simulink model "electric_vehicle3"  (R2018a)
settings: Solver=VariableStepAuto  StartTime=0.0  StopTime=2474  RelTol=1e-3
undefined symbols (not defined in the file): DiscIntNeverNeededParam
libraries: fl_lib x13, nesl_utility x7, sdl_lib x5, elec_lib x3, autolibshared x2, pe_lib x1
settings Model: Creator=Asus  LastModifiedBy=Asus

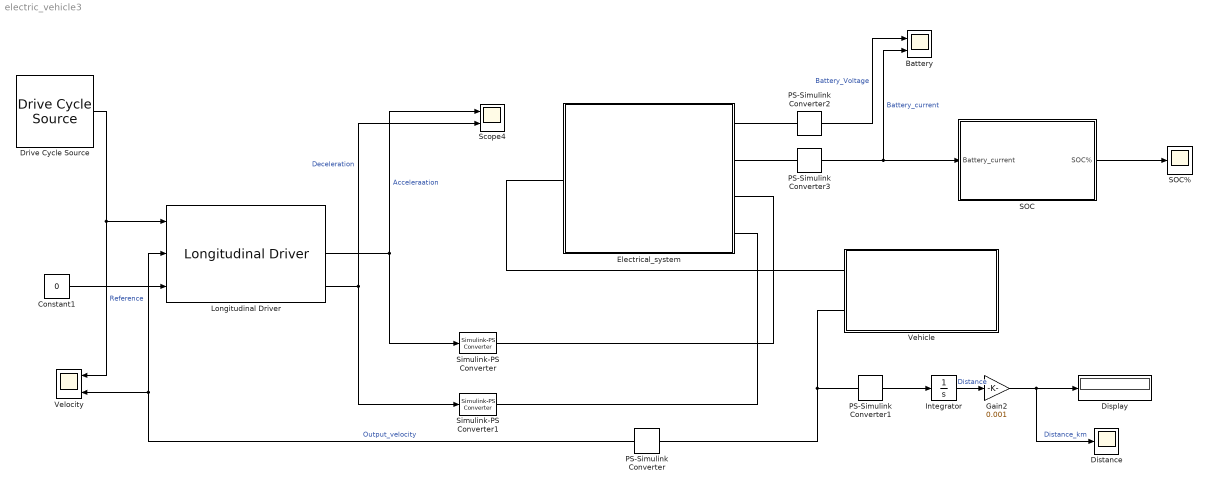
== system electric_vehicle3 ==
  Battery : Scope  NumInputPorts=2
  Constant1 : Constant  Value=0
  Display : Display
  Distance : Scope
  Drive Cycle Source : autolibshared/Drive Cycle Source  cycleVar=FTP75  fileVar=cycleFTP75.mat  tfinal="2474  seconds"  cycleRepeat=off  outAccPort=off  outGearPort=off  gearList=No gear data  t_wot1=5  xdot_woto=0  xdot_wot1=30  t_wot2=20  xdot_wot2=0  t_wotend=30  srcUnit=m/s  outUnit=m/s  srcAccUnit=m/s/s  outAccUnit=m/s^2  dt=0  aMode=1
      settings: SourceProductName=Powertrain Blockset  SourceProductBaseCode=PW
  Electrical_system : Subsystem
  Gain2 : Gain  Gain=0.001
  Integrator : Integrator
  Longitudinal Driver : autolibshared/Longitudinal Driver  aMode=1  vnom=(1500*2*pi*.2286)/60  Kp=40  Ki=1.1  Kaw=0.1  Kff=0.05  Kg=0.01  tauerr=0.03
      settings: SourceProductName=Powertrain Blockset  SourceProductBaseCode=PW
  PS-Simulink Converter : nesl_utility/PS-Simulink Converter  PhysicalDomain=network_engine_domain  SubClassName=ps_output  LeftPortType=input  RightPortType=output  PseudoPeriodic=off  Frequencies=[]  Unit=m/s  AffineConversion=off
  PS-Simulink Converter1 : nesl_utility/PS-Simulink Converter  PhysicalDomain=network_engine_domain  SubClassName=ps_output  LeftPortType=input  RightPortType=output  PseudoPeriodic=off  Frequencies=[]  Unit=m/s  AffineConversion=off
  PS-Simulink Converter2 : nesl_utility/PS-Simulink Converter  PhysicalDomain=network_engine_domain  SubClassName=ps_output  LeftPortType=input  RightPortType=output  PseudoPeriodic=off  Frequencies=[]  Unit=V  AffineConversion=off
  PS-Simulink Converter3 : nesl_utility/PS-Simulink Converter  PhysicalDomain=network_engine_domain  SubClassName=ps_output  LeftPortType=input  RightPortType=output  PseudoPeriodic=off  Frequencies=[]  Unit=A  AffineConversion=off
  SOC : Subsystem
  SOC% : Scope
  Scope4 : Scope  NumInputPorts=2
  Simulink-PS Converter : nesl_utility/Simulink-PS Converter  PhysicalDomain=network_engine_domain  SubClassName=ps_input  LeftPortType=input  RightPortType=output  PseudoPeriodic=off  Frequencies=[]  NoiseDistribution=none  NoiseParameters=[]  Unit=1  AffineConversion=off  FilteringAndDerivatives=provide  SimscapeFilterOrder=1  InputFilterTimeConstant=0.001  UdotUserProvided=0
  Simulink-PS Converter1 : nesl_utility/Simulink-PS Converter  PhysicalDomain=network_engine_domain  SubClassName=ps_input  LeftPortType=input  RightPortType=output  PseudoPeriodic=off  Frequencies=[]  NoiseDistribution=none  NoiseParameters=[]  Unit=1  AffineConversion=off  FilteringAndDerivatives=provide  SimscapeFilterOrder=1  InputFilterTimeConstant=0.001  UdotUserProvided=0
  "Vehicle " : Subsystem
  "Velocity " : Scope  NumInputPorts=2
  wires:
  Drive Cycle Source/1 -> "Velocity "/1, Longitudinal Driver/1  "Reference"
  Longitudinal Driver/2 -> Simulink-PS Converter/1, Scope4/1  "Acceleraation"
  Longitudinal Driver/3 -> Simulink-PS Converter1/1, Scope4/2  "Deceleration"
  PS-Simulink Converter/1 -> Longitudinal Driver/2, "Velocity "/2  "Output_velocity"
  PS-Simulink Converter1/1 -> Integrator/1
  Integrator/1 -> Gain2/1  "Distance"
  PS-Simulink Converter3/1 -> Battery/2, SOC/1(Battery_current)  "Battery_current"
  PS-Simulink Converter2/1 -> Battery/1  "Battery_Voltage"
  Gain2/1 -> Display/1, Distance/1  "Distance_km"
  Constant1/1 -> Longitudinal Driver/3
  SOC/1(SOC%) -> SOC%/1
  connections:
  PS-Simulink Converter/LConn1 -- PS-Simulink Converter1/LConn1 -- "Vehicle "/LConn2
  Electrical_system/RConn1 -- PS-Simulink Converter2/LConn1
  PS-Simulink Converter3/LConn1 -- Electrical_system/RConn2
  Electrical_system/LConn1 -- "Vehicle "/LConn1
  Simulink-PS Converter/RConn1 -- Electrical_system/RConn3
  Simulink-PS Converter1/RConn1 -- Electrical_system/RConn4

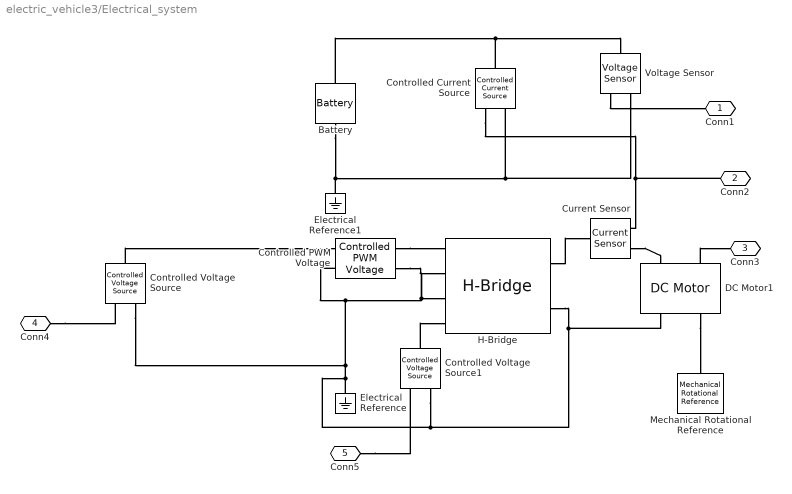
== system electric_vehicle3/Electrical_system ==
  Battery : pe_lib/Sources/Battery  Vnom=24 V  R1=2 Ohm  prm_AH=2  AH=80 hr*A  V1=11.5 V  AH1=25 hr*A  prm_R2=2  R2=2000 Ohm  prm_dyn=1  Rp1=0.005 Ohm  tau1=30 s  Rp2=0.005 Ohm  tau2=30 s  prm_fade=1  N_fade=100  AH_fade=45 hr*A  R1_fade=2.02 Ohm  V1_fade=10.35 V  i_specify=off  i_priority=None  i=0 A  i_nominal_specify=off  i_nominal_unit=A  i_nominal_value=1  v_specify=off  v_priority=None  v=0 V  v_nominal_specify=off  v_nominal_unit=V  v_nominal_value=1  charge_specify=on  charge_priority=High  charge=80 hr*A  charge_nominal_specify=off  charge_nominal_unit=hr*A  charge_nominal_value=1  num_cycles_specify=off  num_cycles_priority=High  num_cycles=0  num_cycles_nominal_specify=off  num_cycles_nominal_unit=1  num_cycles_nominal_value=1  thermal_mass=30000 J/K  Tmeas=298.15 K  Vnom_T2=12 V  R1_T2=2.2 Ohm  V1_T2=11.4 V  R2_T2=2200 Ohm  Rp1_T2=0.005 Ohm  tau1_T2=30 s  Rp2_T2=0.005 Ohm  tau2_T2=30 s  Tmeas2=273.15 K  temperature_specify=off  temperature_priority=High  temperature=298.15 K  temperature_nominal_specify=off  temperature_nominal_unit=K  temperature_nominal_value=1
      settings: SourceProductName=Simscape Power Systems  SourceProductBaseCode=PS
  Controlled Current Source : fl_lib/Electrical/Electrical Sources/Controlled Current Source
  Controlled PWM Voltage : elec_lib/Actuators & Drivers/Drivers/Controlled PWM Voltage  F=50 Hz  TD=0 s  pulse_width_offset=0 s  pulse_min=0 s  Vmin=0 V  Vmax=5 V  Vm=5 V  pwm_or_av=2  event_type=1  sample_time=1e-6 s  u_min=0  u_max=1
      settings: SourceProductName=Simscape Electronics  SourceProductBaseCode=SN
  Controlled Voltage Source : fl_lib/Electrical/Electrical Sources/Controlled Voltage Source
  Controlled Voltage Source1 : fl_lib/Electrical/Electrical Sources/Controlled Voltage Source
  Current Sensor : fl_lib/Electrical/Electrical Sensors/Current Sensor
  DC Motor1 : elec_lib/Actuators & Drivers/Rotational Actuators/DC Motor  parameterization=3  Ra=3.9 Ohm  La=12e-6 H  emf_or_torque=2  Kv=0.072e-3 V/rpm  Ki=6.876e-4 N*m/A  T_stall=0.24e-3 N*m  w_max=19100 rpm  w_rated=15000 rpm  P_rated=0.08 W  V_rated=12 V  J=0.01 g*cm^2  lam_param=1  lam=0 N*m/(rad/s)  i_noload=0 A  V_i_noload=1.5 V  speed0=0 rpm  alpha=3.93e-3 1/K  Tmeas=25 degC  thermal_mass=100 J/K  initial_temperature=25 degC
  Electrical Reference : fl_lib/Electrical/Electrical Elements/Electrical Reference
  Electrical Reference1 : fl_lib/Electrical/Electrical Elements/Electrical Reference
  H-Bridge : elec_lib/Actuators & Drivers/Drivers/H-Bridge  Venable=2.5 V  Vmax=5.0 V  Vreverse=2.5 V  Vbrake=2.5 V  Vm=400 kV  pwm_or_av=2  discontinuous=0  freewheeling_mode=1  freewheeling_mode_disc=3  Ron=0.1 Ohm  Don=0.05 Ohm  Rload=10 Ohm  Lload=1e-5 H  F=10 kHz  thermal_mass=100 J/K  initial_temperature=298.15 K  Ron2=0.1 Ohm  Don2=0.05 Ohm  Tmeas=298.15 K  Tmeas2=398.15 K
      settings: SourceProductName=Simscape Electronics  SourceProductBaseCode=SN
  Mechanical Rotational Reference : fl_lib/Mechanical/Rotational Elements/Mechanical Rotational Reference
  Voltage Sensor : fl_lib/Electrical/Electrical Sensors/Voltage Sensor
  Conn1 : PMIOPort  Side=Right
  Conn2 : PMIOPort  Port=2  Side=Right
  Conn3 : PMIOPort  Port=3  Side=Left
  Conn4 : PMIOPort  Port=4  Side=Right
  Conn5 : PMIOPort  Port=5  Side=Right
  connections:
  Controlled Current Source/RConn1 -- Conn2/RConn1 -- Current Sensor/RConn1
  DC Motor1/RConn2 -- Mechanical Rotational Reference/LConn1
  H-Bridge/RConn2 -- DC Motor1/RConn1 -- Controlled Voltage Source/RConn2 -- Controlled PWM Voltage/RConn2 -- H-Bridge/LConn2 -- H-Bridge/LConn3 -- Controlled PWM Voltage/LConn2 -- Electrical Reference/LConn1 -- Controlled Voltage Source1/RConn2
  Electrical Reference1/LConn1 -- Battery/RConn1 -- Voltage Sensor/RConn2 -- Controlled Current Source/RConn2
  H-Bridge/RConn1 -- Current Sensor/LConn1
  Controlled PWM Voltage/RConn1 -- H-Bridge/LConn1
  Controlled Current Source/LConn1 -- Battery/LConn1 -- Voltage Sensor/LConn1
  Controlled Voltage Source1/LConn1 -- H-Bridge/LConn4
  Controlled Voltage Source/LConn1 -- Controlled PWM Voltage/LConn1
  Conn4/RConn1 -- Controlled Voltage Source/RConn1
  Conn5/RConn1 -- Controlled Voltage Source1/RConn1
  Voltage Sensor/RConn1 -- Conn1/RConn1
  DC Motor1/LConn2 -- Conn3/RConn1
  Current Sensor/RConn2 -- DC Motor1/LConn1

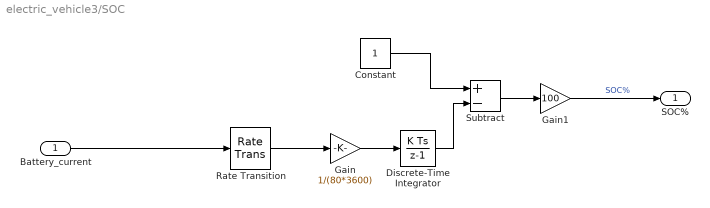
== system electric_vehicle3/SOC ==
  Battery_current : Inport
  Constant : Constant
  Discrete-Time Integrator : DiscreteIntegrator  SampleTime=-1  ICPrevOutput=DiscIntNeverNeededParam  ICPrevScaledInput=DiscIntNeverNeededParam
  Gain : Gain  Gain=1/(80*3600)
  Gain1 : Gain  Gain=100
  Rate Transition : RateTransition
  Subtract : Sum  Inputs=+-
  SOC% : Outport
  wires:
  Subtract/1 -> Gain1/1
  Battery_current/1 -> Rate Transition/1
  Gain/1 -> Discrete-Time Integrator/1
  Constant/1 -> Subtract/1
  Rate Transition/1 -> Gain/1
  Gain1/1 -> SOC%/1  "SOC%"
  Discrete-Time Integrator/1 -> Subtract/2

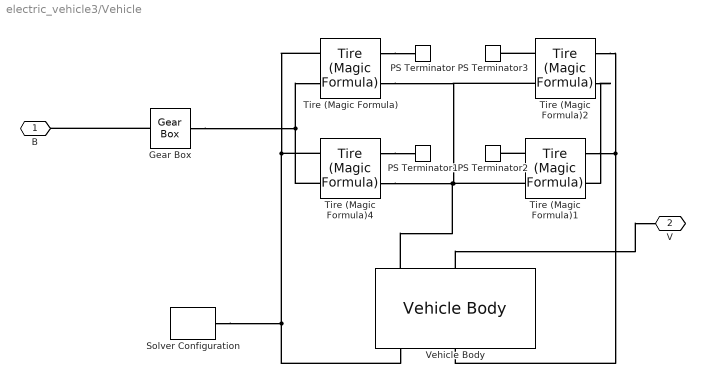
== system electric_vehicle3/Vehicle  ==
  Gear Box : fl_lib/Mechanical/Mechanisms/Gear Box  ratio=5000  t_in_specify=off  t_in_priority=None  t_in=0 N*m  t_in_nominal_specify=off  t_in_nominal_unit=N*m  t_in_nominal_value=1  t_out_specify=off  t_out_priority=None  t_out=0 N*m  t_out_nominal_specify=off  t_out_nominal_unit=N*m  t_out_nominal_value=1
  PS Terminator{,1..3} (4 alike) : fl_lib/Physical Signals/Sinks/PS Terminator
      settings: SourceProductName=Simscape
  Solver Configuration : nesl_utility/Solver Configuration  PhysicalDomain=network_engine_domain  SubClassName=solver  LeftPortType=input  RightPortType=generic  Tones=[]  Harmonics=[]  SimulateNoise=off  Profile=off  UseLocalSampling=off  EnableSwitchedLinearOptims=on  FrequencyDomain=off  UseCCode=off  RelTol=0.001  AbsTol=1e-06  MinStep=1e-09  ToWorkspace=off  RevertToSquareIcSolve=off  NumHomotopyIterations=100  PhasorMode=off  PhasorModeNumHarmonics=1  DoDC=off  ResidualTolerance=1e-09  UseLocalSolver=off  LocalSolverChoice=NE_BACKWARD_EULER_ADVANCER  LocalSolverSampleTime=0.001  DoFixedCost=off  MaxNonlinIter=3  MaxModeIter=2  LinearAlgebra=Sparse  EquationFormulation=NE_TIME_EF  DelaysMemoryBudget=1024  AutomaticFiltering=on  FilteringTimeConstant=0.001
  Tire (Magic Formula){,1..2,4} (4 alike) : sdl_lib/Tires & Vehicles/Tire (Magic Formula)  parameterization=2  F_z1=3000 N  F_x1=3500 N  kappa1=10  B_m=10  C_m=1.9  D_m=1  E_m=0.97  fz0=4000 N  p_Cx=1.685  p_Dx=[1.21, -.037]  p_Ex=[.344, .095, -.02, 0]  p_Kx=[21.51, -.163, .245]  p_Hx=[-.002, .002]  p_Vx=[0, 0]  v_tr_thr=0.1 m/s  r_e=9 in  model_compliance=0  stiffness=1e6 N/m  damping=1000 N/(m/s)  model_inertia=1  inertia=0.001 kg*m^2  initial_velocity=0 rad/s  model_resistance=1  resistance_model=1  coeff=0.005  p_tire=250e3 Pa  alpha=-0.003  beta=0.97  coeff_a=84e-4  coeff_b=6.2e-4 s/m  coeff_c=1.6e-4 s^2/m^2  v_thr=0.001 m/s
      settings: SourceProductName=Simscape Driveline
  Vehicle Body : sdl_lib/Tires & Vehicles/Vehicle Body  mass=80+237 kg  n_w=2  x_f=1520 mm  x_r=1400 mm  y_c=254 mm  model_pitch=0  inertia=4000 kg*m^2  suspension_model=1  k_f=1e4 N/m  b_f=1e4 N/(m/s)  k_r=1e4 N/m  b_r=1e4 N/(m/s)  k_f_TLU=[-2000, -1000, 0, 1000, 2000] N  x_f_TLU=[-.4, -.2, 0, .2, .4] m  b_f_TLU=[-200, -100, 0, 100, 200] N  v_f_TLU=[-4, -2, 0, 2, 4] m/s  k_r_TLU=[-2000, -1000, 0, 1000, 2000] N  x_r_TLU=[-.4, -.2, 0, .2, .4] m  b_r_TLU=[-200, -100, 0, 100, 200] N  v_r_TLU=[-4, -2, 0, 2, 4] m/s  interp_method=simscape.enum.interpolation.linear  extrap_method=simscape.enum.extrapolation.linear  model_hardstop=0  upper_bound_f=.25 m  lower_bound_f=-.25 m  stop_k_f=1e6 N/m  stop_b_f=150 N/(m/s)  upper_bound_r=.25 m  lower_bound_r=-.25 m  stop_k_r=1e6 N/m  stop_b_r=150 N/(m/s)  initial_pitch=0 rad  initial_pitch_rate=0 rad/s  g=9.81 m/s^2  liftoff_warning=0  area=1.33 m^2  Cd=1.2  rho=1.18 kg/m^3  v_specify=off  v_priority=High  v=0 m/s  v_nominal_specify=off  v_nominal_unit=m/s  v_nominal_value=1
      settings: SourceProductName=Simscape Driveline
  B : PMIOPort  Side=Left
  V : PMIOPort  Port=2  Side=Left
  connections:
  Tire (Magic Formula)4/LConn2 -- Gear Box/RConn1 -- Tire (Magic Formula)/LConn2
  Vehicle Body/LConn1 -- Tire (Magic Formula)4/RConn2 -- Tire (Magic Formula)1/RConn2 -- Tire (Magic Formula)2/RConn2 -- Tire (Magic Formula)/RConn2
  Tire (Magic Formula)1/LConn1 -- Tire (Magic Formula)2/LConn1 -- Vehicle Body/RConn2
  Gear Box/LConn1 -- B/RConn1
  Vehicle Body/RConn1 -- Solver Configuration/RConn1 -- Tire (Magic Formula)4/LConn1 -- Tire (Magic Formula)/LConn1
  Tire (Magic Formula)/RConn1 -- PS Terminator/LConn1
  Tire (Magic Formula)4/RConn1 -- PS Terminator1/LConn1
  Tire (Magic Formula)2/RConn1 -- PS Terminator3/LConn1
  Tire (Magic Formula)1/RConn1 -- PS Terminator2/LConn1
  Tire (Magic Formula)2/LConn2 -- Tire (Magic Formula)1/LConn2
  Vehicle Body/LConn2 -- V/RConn1
